simulink model "caiyang"  (R2015b)
settings: Solver=VariableStepAuto  StartTime=0.0  StopTime=10.0  FixedStep=0.05  RelTol=1e-3
libraries: simulink x2
settings Model: Creator=DELL  LastModifiedBy=DELL

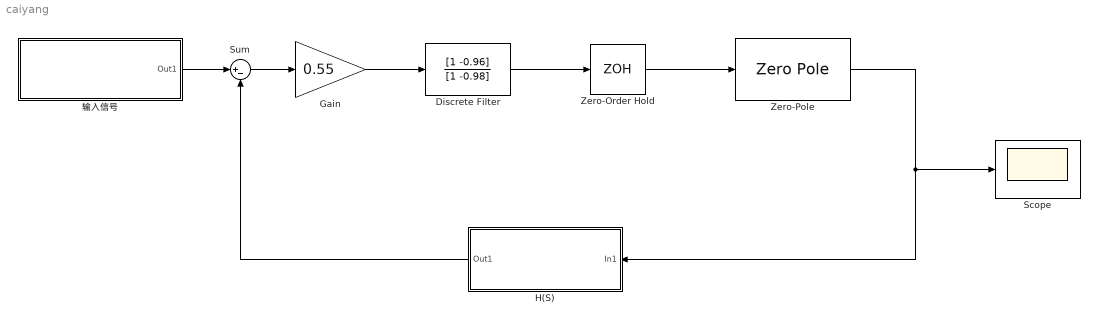
== system caiyang ==
  Discrete Filter : DiscreteFilter  Numerator=[1 -0.96]  Denominator=[1 -0.98]  SampleTime=0.05
  Gain : Gain  Gain=0.55
  H(S) : Subsystem  mask{K2=1, den_h=[0 0 1]}
      mask prompts: K2 "K"; den_h "参数设置"
      mask DialogControl DescTextVar Prompt: H(S)分子参数设置
      mask DialogControl Control2 Prompt: H(S)分母参数设置
      mask Display: dpoly([0 0 K2], den_h, 's')
  Scope : Scope
  Sum : Sum  Inputs=|+-
  Zero-Order Hold : ZeroOrderHold  SampleTime=0.05
  Zero-Pole : ZeroPole  Zeros=[]  Poles=[0 -10 -2]  Gain=[30]
  输入信号 : Subsystem  mask{input_num=阶跃信号, step_time=0, step_init=0, step_final=10}
      mask prompts: input_num "信号输入选择"; step_time "阶跃时间"; step_init "初值"; step_final "终值"
      mask TypeOptions input_num: 阶跃信号 | 斜坡信号 | 加速度信号 | 正弦信号
      mask DialogControl Control1 Prompt: 阶跃信号参数设置
      mask Display:
      | if input_num==1
      |     disp('阶跃输入');
      | elseif input_num==2
      |     disp('斜坡（速度）输入');
      | elseif input_num==3
      |     disp('加速度输入');
      | elseif input_num==4
      |     disp('正弦');
      | else
      |     disp('输入信号选择');
      | end
  wires:
  输入信号/1(Out1) -> Sum/1
  Zero-Pole/1 -> H(S)/1(In1), Scope/1
  H(S)/1(Out1) -> Sum/2
  Sum/1 -> Gain/1
  Gain/1 -> Discrete Filter/1
  Discrete Filter/1 -> Zero-Order Hold/1
  Zero-Order Hold/1 -> Zero-Pole/1

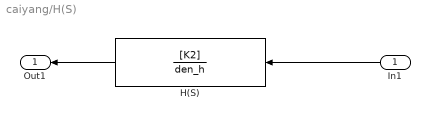
== system caiyang/H(S) ==
  In1 : Inport
  H(S) : TransferFcn  Numerator=[K2]  Denominator=den_h  mask{K2=1, den_h=[0 0 0 1]}
      mask prompts: K2 "K"; den_h "参数输入"
      mask Display: dpoly([0 0 K2], den_h, 's')
  Out1 : Outport
  wires:
  In1/1 -> H(S)/1
  H(S)/1 -> Out1/1

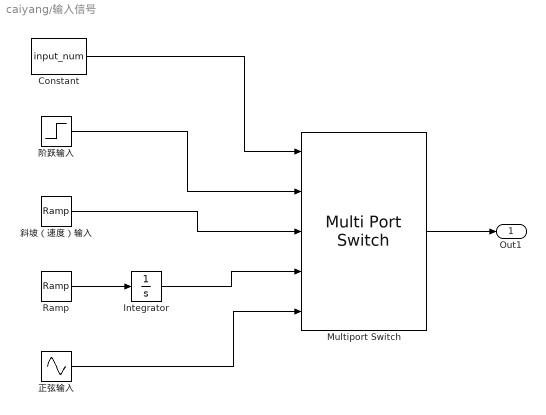
== system caiyang/输入信号 ==
  Constant : Constant  Value=input_num
  Integrator : Integrator
  Multiport Switch : MultiPortSwitch  Inputs=4
  Ramp : simulink/Sources/Ramp  slope=1  start=0  X0=0
  斜坡（速度）输入 : simulink/Sources/Ramp  slope=1  start=0  X0=0
  正弦输入 : Sin  SampleTime=0
  阶跃输入 : Step  Time=step_time  Before=step_init  After=step_final  SampleTime=0
  Out1 : Outport
  wires:
  Ramp/1 -> Integrator/1
  阶跃输入/1 -> Multiport Switch/2
  斜坡（速度）输入/1 -> Multiport Switch/3
  Integrator/1 -> Multiport Switch/4
  Multiport Switch/1 -> Out1/1
  正弦输入/1 -> Multiport Switch/5
  Constant/1 -> Multiport Switch/1
